simulink model "integrated_vehicle_control"  (R2025b)
settings: Solver=VariableStepAuto  StartTime=0.0  StopTime=14  RelTol=1e-3
StopFcn:
  | plot_integrated_results;
values from neighbouring files (symbols this model uses):
  delta_max = deg2rad(30)    [load_parameters.m]    (also in stanley_lateral_control.m)
  k_gain = 1.5    [load_parameters.m]    (also in stanley_lateral_control.m)
  k_soft = 1.0    (= 1)    [load_parameters.m]    (also in stanley_lateral_control.m)
  L = 2.5    [load_parameters.m]    (also in stanley_lateral_control.m)
  theta_path = atan2(diff(y_path), diff(x_path))    [load_parameters.m]    (also in stanley_lateral_control.m)
  x_path = linspace(0, 260, 7000)    [load_parameters.m]    (also in plot_integrated_results.m; stanley_lateral_control.m = linspace(0, 100, 4000))
  y_path = (dy1/2)*(1+tanh(z1)) - (dy2/2)*(1+tanh(z2))    [load_parameters.m]    (also in plot_integrated_results.m; stanley_lateral_control.m)
settings Model: Creator=Biggio  LastModifiedBy=Biggio
settings DataIOCC: ReturnWorkspaceOutputs=off

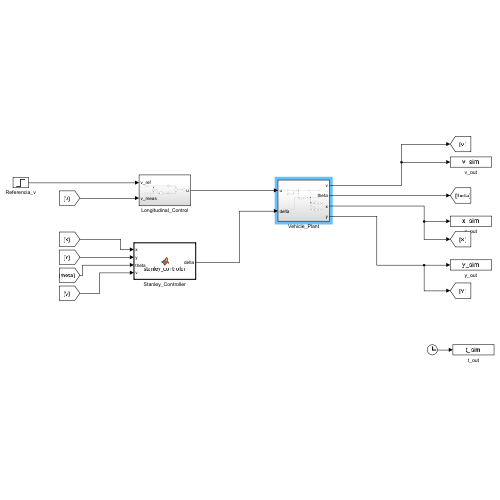
[thumbnail: Simulink's stored preview of the top-level diagram]
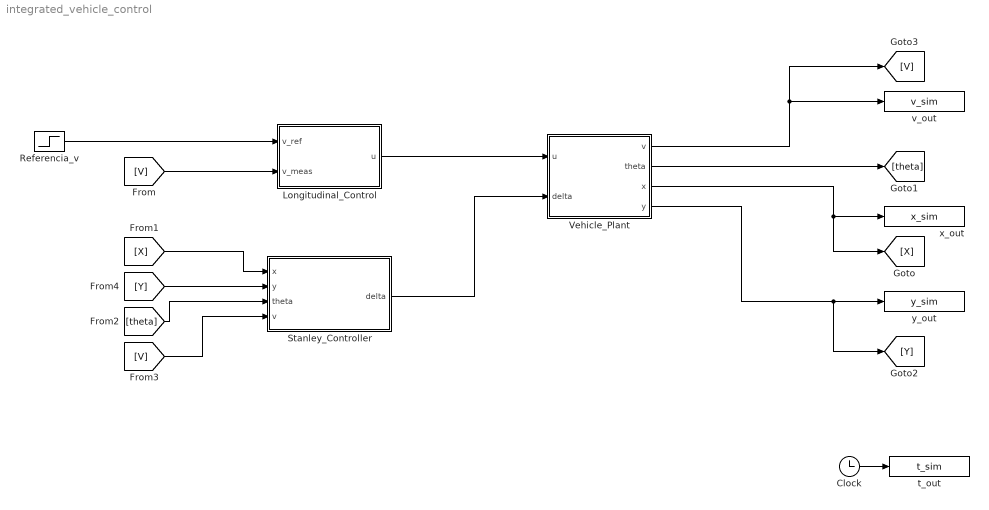
== system integrated_vehicle_control ==
  Clock : Clock
  Longitudinal_Control : Subsystem
  Referencia_v : Step  After=15  SampleTime=0
  Stanley_Controller : MATLAB Function  TreatAsAtomicUnit=on
  Vehicle_Plant : Subsystem
  t_out : ToWorkspace  VariableName=t_sim  SampleTime=-1
  v_out : ToWorkspace  VariableName=v_sim  SampleTime=-1
  x_out : ToWorkspace  VariableName=x_sim  SampleTime=-1
  y_out : ToWorkspace  VariableName=y_sim  SampleTime=-1
  wires:
  Referencia_v/1 -> Longitudinal_Control/1(v_ref)
  Longitudinal_Control/1(u) -> Vehicle_Plant/1(u)
  Vehicle_Plant/1(v) -> [V], v_out/1
  Vehicle_Plant/2(theta) -> [theta]
  Vehicle_Plant/3(x) -> [X], x_out/1
  Vehicle_Plant/4(y) -> [Y], y_out/1
  Stanley_Controller/1(delta) -> Vehicle_Plant/2(delta)
  Clock/1 -> t_out/1
  [V] -> Longitudinal_Control/2(v_meas)
  [X] -> Stanley_Controller/1(x)
  [V] -> Stanley_Controller/4(v)
  [theta] -> Stanley_Controller/3(theta)
  [Y] -> Stanley_Controller/2(y)

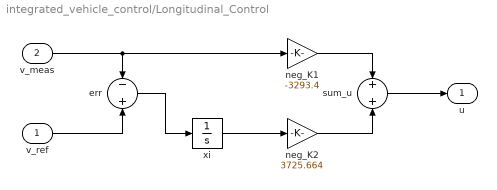
== system integrated_vehicle_control/Longitudinal_Control ==
  v_ref : Inport
  v_meas : Inport  Port=2
  err : Sum  Inputs=-+
  neg_K1 : Gain  Gain=-3293.4
  neg_K2 : Gain  Gain=3725.664
  sum_u : Sum
  xi : Integrator
  u : Outport
  wires:
  v_ref/1 -> err/2
  v_meas/1 -> err/1, neg_K1/1
  err/1 -> xi/1
  xi/1 -> neg_K2/1
  neg_K1/1 -> sum_u/1
  neg_K2/1 -> sum_u/2
  sum_u/1 -> u/1

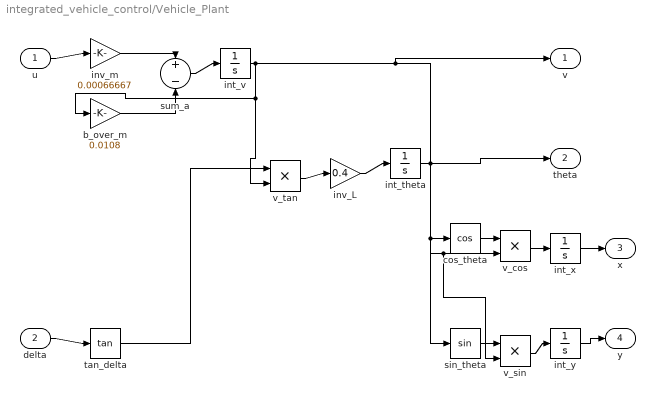
== system integrated_vehicle_control/Vehicle_Plant ==
  u : Inport
  delta : Inport  Port=2
  b_over_m : Gain  Gain=0.0108
  cos_theta : Trigonometry  Operator=cos
  int_theta : Integrator
  int_v : Integrator
  int_x : Integrator
  int_y : Integrator
  inv_L : Gain  Gain=0.4
  inv_m : Gain  Gain=0.00066667
  sin_theta : Trigonometry
  sum_a : Sum  Inputs=+-
  tan_delta : Trigonometry  Operator=tan
  v_cos : Product
  v_sin : Product
  v_tan : Product
  v : Outport
  theta : Outport  Port=2
  x : Outport  Port=3
  y : Outport  Port=4
  wires:
  u/1 -> inv_m/1
  inv_m/1 -> sum_a/1
  int_v/1 -> b_over_m/1, v_tan/2, v_sin/2, v_cos/2, v/1
  b_over_m/1 -> sum_a/2
  sum_a/1 -> int_v/1
  delta/1 -> tan_delta/1
  tan_delta/1 -> v_tan/1
  v_tan/1 -> inv_L/1
  inv_L/1 -> int_theta/1
  int_theta/1 -> sin_theta/1, cos_theta/1, theta/1
  cos_theta/1 -> v_cos/1
  sin_theta/1 -> v_sin/1
  v_cos/1 -> int_x/1
  v_sin/1 -> int_y/1
  int_x/1 -> x/1
  int_y/1 -> y/1

== matlab function integrated_vehicle_control/Stanley_Controller ==
  data: x input; delta output; y input; theta input; v input; x_path parameter; y_path parameter; L parameter; theta_path parameter; k_gain parameter; k_soft parameter; delta_max parameter
function delta = stanley_controller(x, y, theta, v, x_path, y_path, L, theta_path, k_gain, k_soft, delta_max)
    dists = (x_path - (x + L*cos(theta))).^2 + (y_path - (y + L*sin(theta))).^2;
    [~, idx] = min(dists);
    xf = x + L*cos(theta); yf = y + L*sin(theta);
    dx = xf - x_path(idx); dy = yf - y_path(idx);
    e = dx*sin(theta) - dy*cos(theta);
    theta_e = theta_path(idx) - theta;
    theta_e = atan2(sin(theta_e), cos(theta_e));
    delta = theta_e + atan2(k_gain*e, v + k_soft);
    delta = max(min(delta, delta_max), -delta_max);
end
